simulink model "inverter_hysteresis_controller"  (R2015a)
settings: Solver=ode45  StartTime=0.0  StopTime=0.06  MaxStep=1/10000  RelTol=1e-3
libraries: powerlib x9
settings Model: Creator=Windows 10  LastModifiedBy=Windows 10

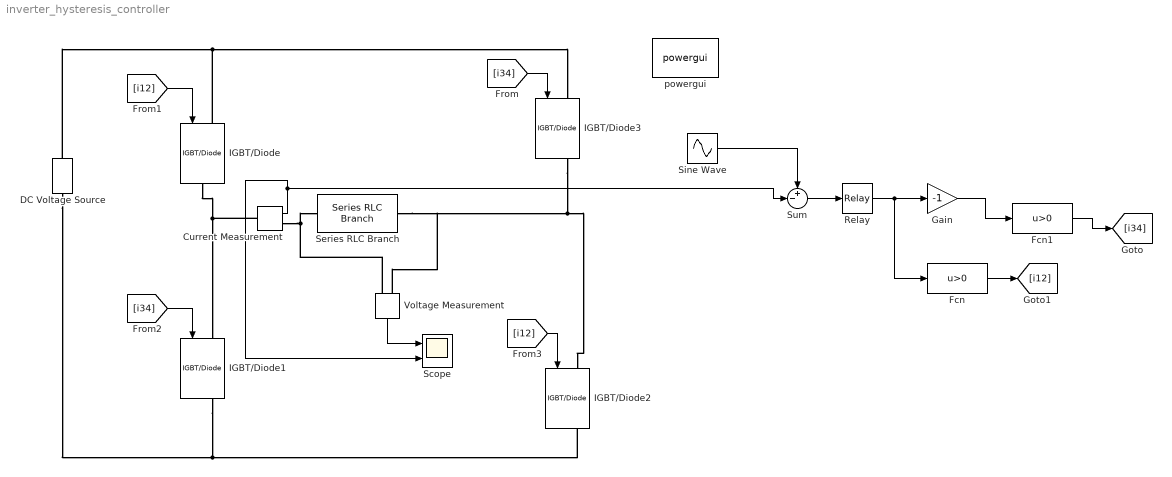
== system inverter_hysteresis_controller ==
  Current Measurement : powerlib/Measurements/Current Measurement  PhasorSimulation=off  OutputType=Complex  PSBequivalent=0
  DC Voltage Source : powerlib/Electrical Sources/DC Voltage Source  Amplitude=200  Measurements=None
  Fcn : Fcn  Expr=u>0
  Fcn1 : Fcn  Expr=u>0
  Gain : Gain  Gain=-1
  IGBT/Diode : powerlib/Power Electronics/IGBT//Diode  Ron=1e-3  Rs=1e5  Cs=inf  Measurements=off
  IGBT/Diode1 : powerlib/Power Electronics/IGBT//Diode  Ron=1e-3  Rs=1e5  Cs=inf  Measurements=on
  IGBT/Diode2 : powerlib/Power Electronics/IGBT//Diode  Ron=1e-3  Rs=1e5  Cs=inf  Measurements=on
  IGBT/Diode3 : powerlib/Power Electronics/IGBT//Diode  Ron=1e-3  Rs=1e5  Cs=inf  Measurements=on
  Relay : Relay  OnSwitchValue=5  OffSwitchValue=-5  OffOutputValue=-1
  Scope : Scope  NumInputPorts=2
      settings: YMin=-5~-5  YMax=5~5
  Series RLC Branch : powerlib/Elements/Series RLC Branch  LConnTagsString=__new0  RConnTagsString=__new0  BranchType=RL  Resistance=2  Inductance=4.8e-3  SetiL0=off  InitialCurrent=0  Capacitance=1e-6  Setx0=off  InitialVoltage=0  Measurements=None
  Sine Wave : Sin  Amplitude=50  Frequency=2*pi*50  SampleTime=0
  Sum : Sum  Inputs=+-|
  Voltage Measurement : powerlib/Measurements/Voltage Measurement  PhasorSimulation=off  OutputType=Complex  PSBequivalent=0
  powergui : powerlib/powergui  Priority=1  SimulationMode=Continuous  SolverType=Tustin/Backward Euler (TBE)  SampleTime=50e-6  frequency=60  SPID=off  DisableSnubberDevices=off  DisableRonSwitches=off  DisableVfSwitches=off  SwTol=0  DisplayEquations=off  Interpol=off  methode=off  Ts=100  FunctionMessages=off  echomessages=off  HookPort=off  EnableUseOfTLC=off  x0status=blocks  frequencyindice=0  Pbase=100e6  ErrMax=1e-4  Iterations=50  UnitsV=kV  UnitsW=MW  buscounter=0  RestoreLinks=warning  ResistiveCurrentMeasurement=off  Frange=[0:2:500]  Ylog=off  Xlog=on  ShowGrid=off  save=off  variable=ZData  structure=0  ZoomFFT=off  StartTime=0.0  cycles=1  DisplayStyle=1  fundamental=60  FreqAxis=off  MaxFrequency=1000  frequencyindicesteady=1  RmsSteady=1  display=off
  wires:
  Voltage Measurement/1 -> Scope/1
  Gain/1 -> Fcn1/1
  Fcn/1 -> [i12]
  Fcn1/1 -> [i34]
  [i12] -> IGBT/Diode/1
  [i12] -> IGBT/Diode2/1
  [i34] -> IGBT/Diode3/1
  [i34] -> IGBT/Diode1/1
  Sine Wave/1 -> Sum/1
  Current Measurement/1 -> Sum/2, Scope/2
  Sum/1 -> Relay/1
  Relay/1 -> Fcn/1, Gain/1
  connections:
  IGBT/Diode/RConn1 -- Current Measurement/LConn1 -- IGBT/Diode1/LConn1
  IGBT/Diode3/RConn1 -- IGBT/Diode2/LConn1 -- Voltage Measurement/LConn2 -- Series RLC Branch/RConn1
  IGBT/Diode1/RConn1 -- DC Voltage Source/LConn1 -- IGBT/Diode2/RConn1
  IGBT/Diode/LConn1 -- IGBT/Diode3/LConn1 -- DC Voltage Source/RConn1
  Current Measurement/RConn1 -- Series RLC Branch/LConn1 -- Voltage Measurement/LConn1
